simulink model "dron_filtro_complementario_version2015"  (R2015b)
settings: Solver=FixedStepDiscrete  StartTime=0.0  StopTime=inf  FixedStep=0.03  RelTol=1e-3
undefined symbols (not defined in the file): DiscIntNeverNeededParam
libraries: simulink x2, RASPlib x2, arduinolib x2
settings Model: SimulationMode=external  ExtModeTrigDuration=2  Creator=jorge  LastModifiedBy=jorge
settings OptimizationCC: OptimizeModelRefInitCode=on  LifeSpan=Inf  MaxStackSize=64
settings HardwareCC: ProdBitPerInt=16  ProdBitPerPointer=16  ProdLargestAtomicFloat=None  ProdWordSize=8  ProdHWDeviceType=Atmel->AVR
settings RTWCC: SystemTargetFile=ert.tlc  TemplateMakefile=ert_default_tmf  Description=Embedded Coder  Toolchain=Arduino AVR v1.6.1  BuildConfiguration=Faster Runs
settings CodeAppCC: IgnoreCustomStorageClasses=off
settings ERTTargetCC: SupportContinuousTime=on  SupportVariableSizeSignals=on  ExtMode=on  ExtModeMexFile=ext_serial_win32_comm_rtt  ExtModeMexArgs=0 5 115200

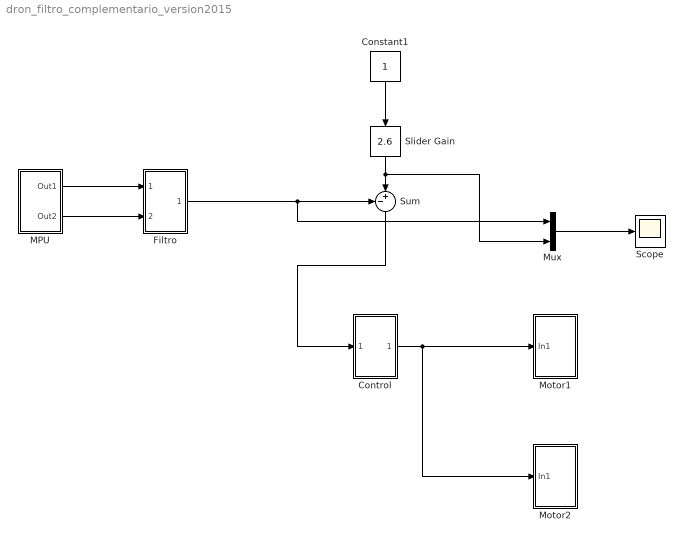
== system dron_filtro_complementario_version2015 ==
  Constant1 : Constant
  Control : Subsystem
  "Filtro " : Subsystem
  "MPU " : Subsystem
  Motor1 : Subsystem
  Motor2 : Subsystem
  Mux : Mux  Inputs=2
  Scope : Scope
  Slider Gain : simulink/Math Operations/Slider Gain  low=-25  gain=2.6  high=35
  Sum : Sum  Inputs=-+|
  wires:
  "MPU "/1(Out1) -> "Filtro "/1(In1)
  "MPU "/2(Out2) -> "Filtro "/2(In2)
  "Filtro "/1(Out3) -> Mux/1, Sum/1
  Mux/1 -> Scope/1
  Sum/1 -> Control/1(In1)
  Control/1(Out1) -> Motor2/1(In1), Motor1/1(In1)
  Constant1/1 -> Slider Gain/1
  Slider Gain/1 -> Mux/2, Sum/2

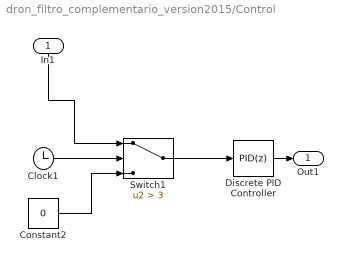
== system dron_filtro_complementario_version2015/Control ==
  In1 : Inport
  Clock1 : Clock
  Constant2 : Constant  Value=0
  Discrete PID Controller : simulink/Continuous/PID Controller  Controller=PID  TimeDomain=Discrete-time  SampleTime=-1  IntegratorMethod=Forward Euler  FilterMethod=Forward Euler  Form=Parallel  UseFilter=on  ControllerParametersSource=internal  P=0.11  I=0.0825  D=0.016  N=30  InitialConditionSource=internal  InitialConditionForIntegrator=0  InitialConditionForFilter=0  ExternalReset=none  LimitOutput=off  UpperSaturationLimit=inf  LowerSaturationLimit=-inf  LinearizeAsGain=off  AntiWindupMode=none  Kb=1  TrackingMode=off  Kt=1  PParamMin=[]  PParamMax=[]  IParamMin=[]  IParamMax=[]  DParamMin=[]  DParamMax=[]  NParamMin=[]  NParamMax=[]  KbParamMin=[]  KbParamMax=[]  KtParamMin=[]  KtParamMax=[]  POutMin=[]  POutMax=[]  IOutMin=[]  IOutMax=[]  DOutMin=[]  DOutMax=[]  NOutMin=[]  NOutMax=[]  KbOutMin=[]  KbOutMax=[]  KtOutMin=[]  KtOutMax=[]  IntegratorOutMin=[]  IntegratorOutMax=[]  FilterOutMin=[]  FilterOutMax=[]  SumOutMin=[]  SumOutMax=[]  SumI1OutMin=[]  SumI1OutMax=[]  SumI2OutMin=[]  SumI2OutMax=[]  SumI3OutMin=[]  SumI3OutMax=[]  SumDOutMin=[]  SumDOutMax=[]  SaturationOutMin=[]  SaturationOutMax=[]  IntegratorContinuousStateAttributes=''  IntegratorStateMustResolveToSignalObject=off  IntegratorRTWStateStorageClass=Auto  FilterContinuousStateAttributes=''  FilterStateMustResolveToSignalObject=off  FilterRTWStateStorageClass=Auto  DifferentiatorICPrevScaledInput=0  DifferentiatorOutMin=[]  DifferentiatorOutMax=[]
  Switch1 : Switch  Criteria=u2 > Threshold  Threshold=3
  Out1 : Outport
  wires:
  Discrete PID Controller/1 -> Out1/1
  Switch1/1 -> Discrete PID Controller/1
  Clock1/1 -> Switch1/2
  Constant2/1 -> Switch1/3
  In1/1 -> Switch1/1

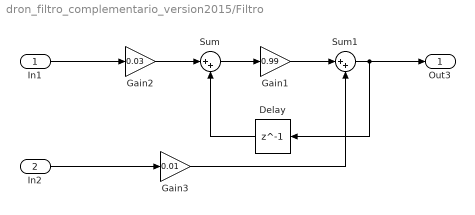
== system dron_filtro_complementario_version2015/Filtro  ==
  In1 : Inport
  In2 : Inport  Port=2
  Delay : Delay  DelayLength=1  InitialCondition=0
  Gain1 : Gain  Gain=0.99
  Gain2 : Gain  Gain=0.03
  Gain3 : Gain  Gain=0.01
  Sum : Sum  Inputs=|++
  Sum1 : Sum  Inputs=|++
  Out3 : Outport
  wires:
  Delay/1 -> Sum/2
  Sum/1 -> Gain1/1
  In2/1 -> Gain3/1
  Gain1/1 -> Sum1/1
  Sum1/1 -> Out3/1, Delay/1
  In1/1 -> Gain2/1
  Gain2/1 -> Sum/1
  Gain3/1 -> Sum1/2

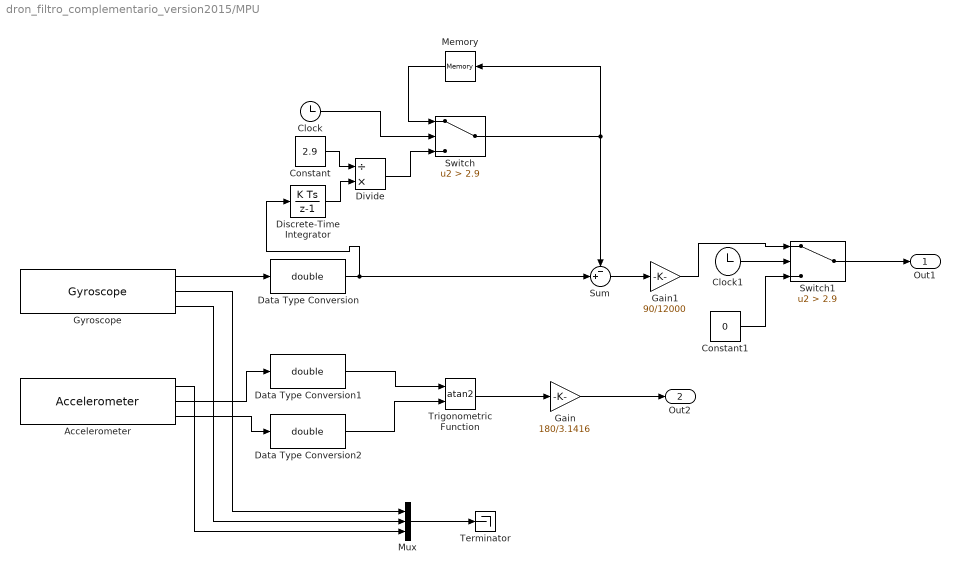
== system dron_filtro_complementario_version2015/MPU  ==
  Accelerometer : RASPlib/Accelerometer  SimulateUsing=Code generation
  Clock : Clock
  Clock1 : Clock
  Constant : Constant  Value=2.9
  Constant1 : Constant  Value=0
  Data Type Conversion : DataTypeConversion  OutDataTypeStr=double
  Data Type Conversion1 : DataTypeConversion  OutDataTypeStr=double
  Data Type Conversion2 : DataTypeConversion  OutDataTypeStr=double
  Discrete-Time Integrator : DiscreteIntegrator  InitialConditionSetting=State (most efficient)  SampleTime=-1  ICPrevOutput=DiscIntNeverNeededParam  ICPrevScaledInput=DiscIntNeverNeededParam
  Divide : Product  Inputs=/*
  Gain : Gain  Gain=180/3.1416
  Gain1 : Gain  Gain=90/12000
  Gyroscope : RASPlib/Gyroscope  DLPFmode=0
  Memory : Memory
  Mux : Mux  Inputs=3
  Sum : Sum  Inputs=-+|
  Switch : Switch  Criteria=u2 > Threshold  Threshold=2.9
  Switch1 : Switch  Criteria=u2 > Threshold  Threshold=2.9
  Terminator : Terminator
  Trigonometric Function : Trigonometry  Operator=atan2
  Out1 : Outport
  Out2 : Outport  Port=2
  wires:
  Clock/1 -> Switch/2
  Gyroscope/3 -> Mux/2
  Switch/1 -> Sum/1, Memory/1
  Sum/1 -> Gain1/1
  Gain/1 -> Out2/1
  Clock1/1 -> Switch1/2
  Switch1/1 -> Out1/1
  Mux/1 -> Terminator/1
  Gyroscope/2 -> Mux/1
  Trigonometric Function/1 -> Gain/1
  Data Type Conversion/1 -> Sum/2, Discrete-Time Integrator/1
  Data Type Conversion1/1 -> Trigonometric Function/1
  Data Type Conversion2/1 -> Trigonometric Function/2
  Constant/1 -> Divide/1
  Discrete-Time Integrator/1 -> Divide/2
  Gyroscope/1 -> Data Type Conversion/1
  Divide/1 -> Switch/3
  Memory/1 -> Switch/1
  Gain1/1 -> Switch1/1
  Constant1/1 -> Switch1/3
  Accelerometer/2 -> Data Type Conversion1/1
  Accelerometer/3 -> Data Type Conversion2/1
  Accelerometer/1 -> Mux/3

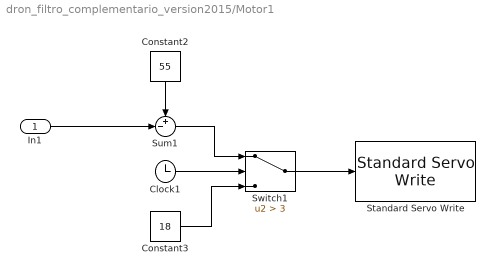
== system dron_filtro_complementario_version2015/Motor1 ==
  In1 : Inport
  Clock1 : Clock
  Constant2 : Constant  Value=55
  Constant3 : Constant  Value=18
  Standard Servo Write : arduinolib/Standard Servo Write  pinNumber=9  blockPlatform=arduino
  Sum1 : Sum  Inputs=+-|
  Switch1 : Switch  Criteria=u2 > Threshold  Threshold=3
  wires:
  In1/1 -> Sum1/2
  Constant2/1 -> Sum1/1
  Constant3/1 -> Switch1/3
  Clock1/1 -> Switch1/2
  Sum1/1 -> Switch1/1
  Switch1/1 -> Standard Servo Write/1

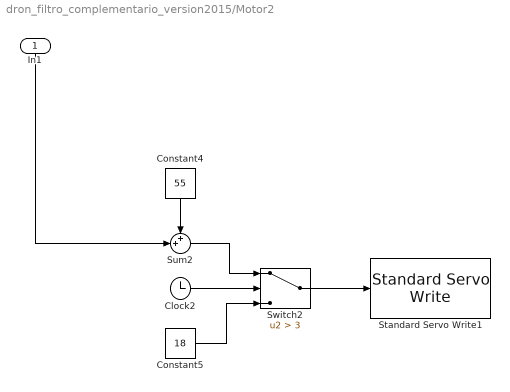
== system dron_filtro_complementario_version2015/Motor2 ==
  In1 : Inport
  Clock2 : Clock
  Constant4 : Constant  Value=55
  Constant5 : Constant  Value=18
  Standard Servo Write1 : arduinolib/Standard Servo Write  pinNumber=10  blockPlatform=arduino
  Sum2 : Sum  Inputs=++|
  Switch2 : Switch  Criteria=u2 > Threshold  Threshold=3
  wires:
  In1/1 -> Sum2/2
  Constant5/1 -> Switch2/3
  Constant4/1 -> Sum2/1
  Switch2/1 -> Standard Servo Write1/1
  Sum2/1 -> Switch2/1
  Clock2/1 -> Switch2/2
